simulink model "DYNctl_ver4_etud_obfusc"  (R2018b)
settings: Solver=ode45  StartTime=0.0  StopTime=tfin  FixedStep=0.001  RelTol=1e-09  EnableMultiTasking=on
undefined symbols (not defined in the file or in its folder): Aplaque, Asphere, Bplaque, Bsphere, Cplaque, Csphere, Dplaque, Dsphere, invTDEF
settings Model: Creator=delafontaine  LastModifiedBy=Vincent
settings DataIOCC: LimitDataPoints=on  SaveFormat=Array  SignalLoggingSaveFormat=ModelDataLogs
settings OptimizationCC: LifeSpan=inf
settings DebuggingCC: UnderspecifiedInitializationDetection=Classic  MergeDetectMultiDrivingBlocksExec=none  MultiTaskDSMMsg=warning  MultiTaskCondExecSysMsg=none  SFUnexpectedBacktrackingDiag=warning  SFNoUnconditionalDefaultTransitionDiag=warning  SFExecutionAtInitializationDiag=none
settings HardwareCC: ProdBitPerPointer=32  ProdBitPerSizeT=32  ProdBitPerPtrDiffT=32  ProdLargestAtomicFloat=None  ProdIntDivRoundTo=Undefined  ProdEndianess=Unspecified  ProdWordSize=32  ProdHWDeviceType=32-bit Generic
settings ModelReferenceCC: PropagateSignalLabelsOutOfModel=off
settings SFSimCC: SimUseLocalCustomCode=off
settings RTWCC: RTWUseLocalCustomCode=off
settings CodeAppCC: StateflowObjectComments=on
settings GRTTargetCC: TargetLangStandard=C89/C90 (ANSI)  GeneratePreprocessorConditionals=Disable all
settings ConfigComp: CovMetricSettings=dw  CovHtmlReporting=on  CovSaveCumulativeToWorkspaceVar=on  CovSaveSingleToWorkspaceVar=on  CovExternalEMLEnable=off  CovSFcnEnable=off

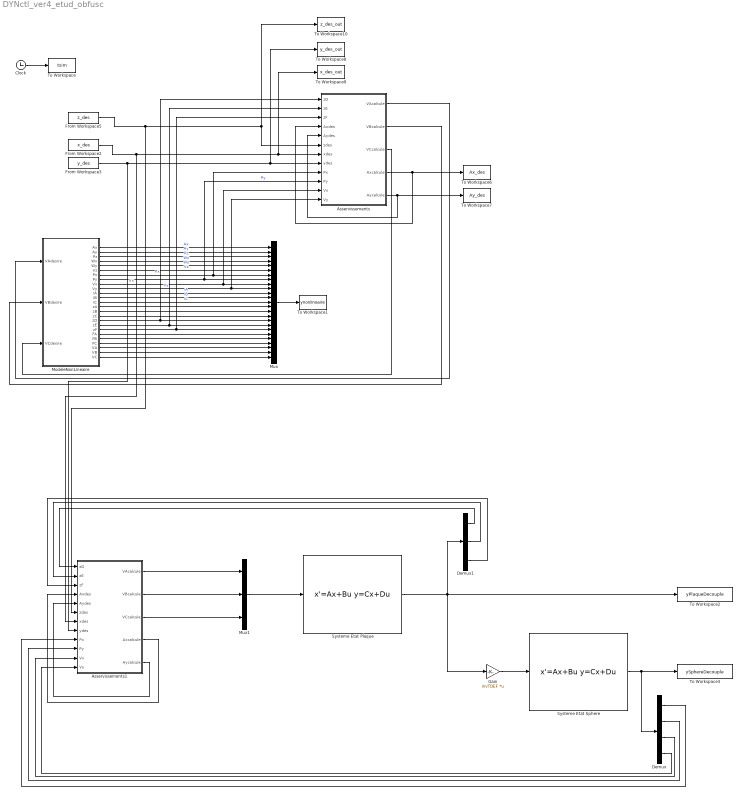
== system DYNctl_ver4_etud_obfusc ==
  Asservissements : Subsystem
      mask help: Simulink:masks:GenSFuncDesc_MD
      mask Help: eval('feval(''rtwprivate'',''rtwhelpview'',''rtw_sfcn_block'')');
  Asservissements1 : Subsystem
      mask help: Simulink:masks:GenSFuncDesc_MD
      mask Help: eval('feval(''rtwprivate'',''rtwhelpview'',''rtw_sfcn_block'')');
  Clock : Clock
  Demux : Demux
  Demux1 : Demux  Outputs=3
  From Workspace2 : FromWorkspace  VariableName=x_des  SampleTime=0  Interpolate=off  OutputAfterFinalValue=Holding final value
  From Workspace3 : FromWorkspace  VariableName=y_des  SampleTime=0  Interpolate=off  OutputAfterFinalValue=Holding final value
  From Workspace5 : FromWorkspace  VariableName=z_des  SampleTime=0  Interpolate=off  OutputAfterFinalValue=Holding final value
  Gain : Gain  Gain=invTDEF  Multiplication=Matrix(K*u)
  ModeleNonLineaire : Subsystem
      mask help: Simulink:masks:GenSFuncDesc_MD
      mask Help: eval('feval(''rtwprivate'',''rtwhelpview'',''rtw_sfcn_block'')');
  Mux : Mux  Inputs=25
  Mux1 : Mux  Inputs=3
  Systeme Etat Plaque : StateSpace  A=Aplaque  B=Bplaque  C=Cplaque  D=Dplaque  InitialCondition=0
  Systeme Etat Sphere : StateSpace  A=Asphere  B=Bsphere  C=Csphere  D=Dsphere  InitialCondition=0
  To Workspace : ToWorkspace  VariableName=tsim  SampleTime=-1
  To Workspace1 : ToWorkspace  VariableName=ynonlineaire  SampleTime=-1
  To Workspace10 : ToWorkspace  VariableName=z_des_out  SampleTime=-1
  To Workspace2 : ToWorkspace  VariableName=yPlaqueDecouple  SaveFormat=Timeseries  SampleTime=-1
  To Workspace3 : ToWorkspace  VariableName=ySphereDecouple  SaveFormat=Timeseries  SampleTime=-1
  To Workspace6 : ToWorkspace  VariableName=Ax_des  SampleTime=-1
  To Workspace7 : ToWorkspace  VariableName=Ay_des  SampleTime=-1
  To Workspace8 : ToWorkspace  VariableName=y_des_out  SampleTime=-1
  To Workspace9 : ToWorkspace  VariableName=x_des_out  SampleTime=-1
  wires:
  Mux/1 -> To Workspace1/1
  Clock/1 -> To Workspace/1
  From Workspace5/1 -> Asservissements1/6(zdes), Asservissements/6(zdes), To Workspace10/1
  ModeleNonLineaire/1(Ax) -> Mux/1  "Ax"
  ModeleNonLineaire/2(Ay) -> Mux/2  "Ay"
  ModeleNonLineaire/3(Pz) -> Mux/3  "Pz"
  ModeleNonLineaire/4(Wx) -> Mux/4  "Wx"
  ModeleNonLineaire/5(Wy) -> Mux/5  "Wy"
  ModeleNonLineaire/6(Vz) -> Mux/6  "Vz"
  ModeleNonLineaire/7(Px) -> Asservissements/9(Px), Mux/7  "Px"
  ModeleNonLineaire/8(Py) -> Asservissements/10(Py), Mux/8  "Py"
  ModeleNonLineaire/9(Vx) -> Asservissements/11(Vx), Mux/9  "Vx"
  ModeleNonLineaire/10(Vy) -> Asservissements/12(Vy), Mux/10  "Vy"
  ModeleNonLineaire/11(IA) -> Mux/11  "IA"
  ModeleNonLineaire/12(IB) -> Mux/12  "IB"
  ModeleNonLineaire/13(IC) -> Mux/13  "IC"
  From Workspace3/1 -> Asservissements1/8(ydes), Asservissements/8(ydes), To Workspace8/1
  From Workspace2/1 -> Asservissements1/7(xdes), Asservissements/7(xdes), To Workspace9/1
  ModeleNonLineaire/20(FA) -> Mux/20
  ModeleNonLineaire/21(FB) -> Mux/21
  ModeleNonLineaire/22(FC) -> Mux/22
  ModeleNonLineaire/23(VA) -> Mux/23
  ModeleNonLineaire/24(VB) -> Mux/24
  ModeleNonLineaire/25(VC) -> Mux/25
  ModeleNonLineaire/17(zD) -> Asservissements/1(zD), Mux/17
  ModeleNonLineaire/18(zE) -> Asservissements/2(zE), Mux/18
  ModeleNonLineaire/19(zF) -> Asservissements/3(zF), Mux/19
  ModeleNonLineaire/14(zA) -> Mux/14
  ModeleNonLineaire/15(zB) -> Mux/15
  ModeleNonLineaire/16(zC) -> Mux/16
  Asservissements/4(Axcalcule) -> Asservissements/4(Axdes), To Workspace6/1
  Asservissements/5(Aycalcule) -> Asservissements/5(Aydes), To Workspace7/1
  Asservissements/1(VAcalcule) -> ModeleNonLineaire/1(VAdesire)
  Asservissements/2(VBcalcule) -> ModeleNonLineaire/2(VBdesire)
  Mux1/1 -> Systeme Etat Plaque/1
  Systeme Etat Plaque/1 -> Demux1/1, Gain/1, To Workspace2/1
  Asservissements/3(VCcalcule) -> ModeleNonLineaire/3(VCdesire)
  Asservissements1/1(VAcalcule) -> Mux1/1
  Asservissements1/2(VBcalcule) -> Mux1/2
  Asservissements1/3(VCcalcule) -> Mux1/3
  Asservissements1/4(Axcalcule) -> Asservissements1/4(Axdes)
  Asservissements1/5(Aycalcule) -> Asservissements1/5(Aydes)
  Gain/1 -> Systeme Etat Sphere/1
  Systeme Etat Sphere/1 -> To Workspace3/1, Demux/1
  Demux/1 -> Asservissements1/9(Px)
  Demux/2 -> Asservissements1/10(Py)
  Demux/3 -> Asservissements1/11(Vx)
  Demux/4 -> Asservissements1/12(Vy)
  Demux1/1 -> Asservissements1/1(zD)
  Demux1/2 -> Asservissements1/2(zE)
  Demux1/3 -> Asservissements1/3(zF)

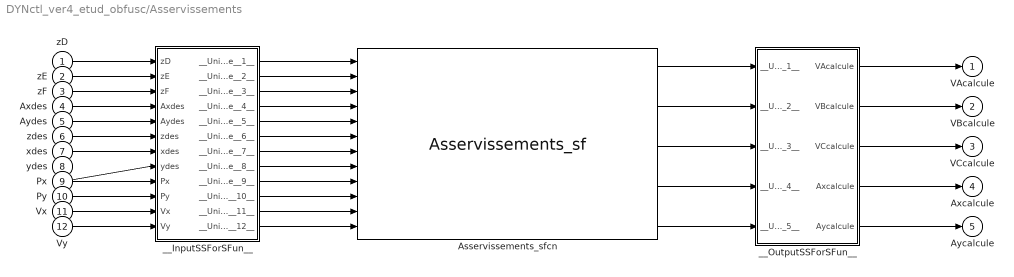
== system DYNctl_ver4_etud_obfusc/Asservissements ==
  zD : Inport
  zE : Inport  Port=2
  zF : Inport  Port=3
  Axdes : Inport  Port=4
  Aydes : Inport  Port=5
  zdes : Inport  Port=6
  xdes : Inport  Port=7
  ydes : Inport  Port=8
  Px : Inport  Port=9
  Py : Inport  Port=10
  Vx : Inport  Port=11
  Vy : Inport  Port=12
  Asservissements_sfcn : S-Function  FunctionName=Asservissements_sf  SFunctionModules=""  SFunctionDeploymentMode=off  EnableBusSupport=off  mask{rtw_sf_name=Asservissements_sf, showVar=off}
      mask prompts: rtw_sf_name "Simulink:masks:GenSFuncName_MP"; showVar "Simulink:masks:GenSFuncShowModuleList_MP"
      mask help: Simulink:masks:GenSFuncDesc_MD
      mask init:
      | displist = '';
      | if ~strcmp(get_param(gcb, 'FunctionName'), rtw_sf_name);
      |   set_param(gcb, 'FunctionName', rtw_sf_name);
      | end
      | % Check if we are generating code
      | rtw_mode = false;
      | if strcmpi(get_param(bdroot(gcb),'SimulationStatus'),'Initializing')
      | 	rtw_mode = strcmpi(get_param(bdroot(gcb),'BuildingRTWCode'),'on') && ...
      | 		~strcmpi(get_param(bdroot(gcb),'TargetStyle'),'SimulationTarget');
      | end
      | if showVar || rtw_mode
      | 	if exist('rtwsfunc') == 2 | exist('rtwsfunc') == 6
      | 		tmplist = rtwsfunc(rtw_sf_name,gcb);
      | 		tmplist = DAStudio.message('Simulink:masks:GenSFuncListOfModules_IC', tmplist);
      | 	elseif showVar
      | 		tmplist1 = DAStudio.message('Simulink:masks:GenSFuncListOfModules_IC', '');
      |         tmplist2 = DAStudio.message('Simulink:masks:GenSFuncNotLicensed_IC');
      |         tmplist = [tmplist1 tmplist2];
      |  	end
      | end
      | if showVar
      |   displist = tmplist;
      | end
      settings: CopyFcn=|
      | if ~strcmp(get_param(gcb,'Linkstatus'),'none') && ...
      | ~strcmp(get_param(gcb,'Linkstatus'),'implicit')
      |   set_param(gcb,'LinkStatus','none');
      | end
      mask Help: eval('feval(''rtwprivate'',''rtwhelpview'',''rtw_sfcn_block'')');
      mask Display:
      | port_label('input',1,'zD');
      | port_label('input',2,'zE');
      | port_label('input',3,'zF');
      | port_label('input',4,'Axdes');
      | port_label('input',5,'Aydes');
      | port_label('input',6,'zdes');
      | port_label('input',7,'xdes');
      | port_label('input',8,'ydes');
      | port_label('input',9,'Px');
      | port_label('input',10,'Py');
      | port_label('input',11,'Vx');
      | port_label('input',12,'Vy');
      | port_label('output',1,'VAcalcule');
      | port_label('output',2,'VBcalcule');
      | port_label('output',3,'VCcalcule');
      | port_label('output',4,'Axcalcule');
      | port_label('output',5,'Aycalcule');
  __InputSSForSFun__ : Subsystem
  __OutputSSForSFun__ : Subsystem
  VAcalcule : Outport
  VBcalcule : Outport  Port=2
  VCcalcule : Outport  Port=3
  Axcalcule : Outport  Port=4
  Aycalcule : Outport  Port=5
  wires:
  zD/1 -> __InputSSForSFun__/1(zD)
  zE/1 -> __InputSSForSFun__/2(zE)
  zF/1 -> __InputSSForSFun__/3(zF)
  Axdes/1 -> __InputSSForSFun__/4(Axdes)
  Aydes/1 -> __InputSSForSFun__/5(Aydes)
  zdes/1 -> __InputSSForSFun__/6(zdes)
  xdes/1 -> __InputSSForSFun__/7(xdes)
  ydes/1 -> __InputSSForSFun__/8(ydes)
  Px/1 -> __InputSSForSFun__/9(Px)
  Py/1 -> __InputSSForSFun__/10(Py)
  Vx/1 -> __InputSSForSFun__/11(Vx)
  Vy/1 -> __InputSSForSFun__/12(Vy)
  __InputSSForSFun__/1(__UniqueOutportName__1__) -> Asservissements_sfcn/1
  __InputSSForSFun__/2(__UniqueOutportName__2__) -> Asservissements_sfcn/2
  __InputSSForSFun__/3(__UniqueOutportName__3__) -> Asservissements_sfcn/3
  __InputSSForSFun__/4(__UniqueOutportName__4__) -> Asservissements_sfcn/4
  __InputSSForSFun__/5(__UniqueOutportName__5__) -> Asservissements_sfcn/5
  __InputSSForSFun__/6(__UniqueOutportName__6__) -> Asservissements_sfcn/6
  __InputSSForSFun__/7(__UniqueOutportName__7__) -> Asservissements_sfcn/7
  __InputSSForSFun__/8(__UniqueOutportName__8__) -> Asservissements_sfcn/8
  __InputSSForSFun__/9(__UniqueOutportName__9__) -> Asservissements_sfcn/9
  __InputSSForSFun__/10(__UniqueOutportName__10__) -> Asservissements_sfcn/10
  __InputSSForSFun__/11(__UniqueOutportName__11__) -> Asservissements_sfcn/11
  __InputSSForSFun__/12(__UniqueOutportName__12__) -> Asservissements_sfcn/12
  Asservissements_sfcn/1 -> __OutputSSForSFun__/1(__UniqueInportName__1__)
  Asservissements_sfcn/2 -> __OutputSSForSFun__/2(__UniqueInportName__2__)
  Asservissements_sfcn/3 -> __OutputSSForSFun__/3(__UniqueInportName__3__)
  Asservissements_sfcn/4 -> __OutputSSForSFun__/4(__UniqueInportName__4__)
  Asservissements_sfcn/5 -> __OutputSSForSFun__/5(__UniqueInportName__5__)
  __OutputSSForSFun__/1(VAcalcule) -> VAcalcule/1
  __OutputSSForSFun__/2(VBcalcule) -> VBcalcule/1
  __OutputSSForSFun__/3(VCcalcule) -> VCcalcule/1
  __OutputSSForSFun__/4(Axcalcule) -> Axcalcule/1
  __OutputSSForSFun__/5(Aycalcule) -> Aycalcule/1

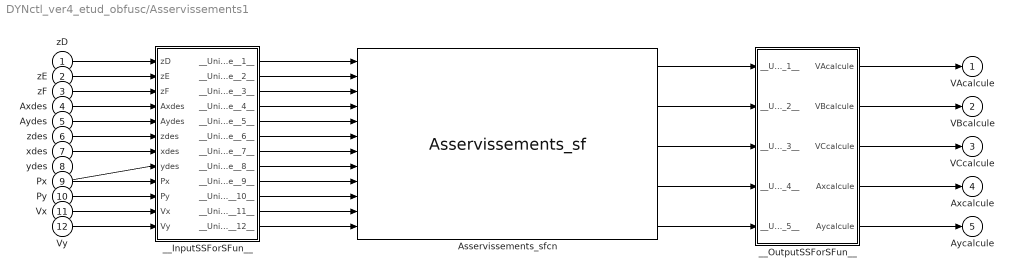
== system DYNctl_ver4_etud_obfusc/Asservissements1 ==
  zD : Inport
  zE : Inport  Port=2
  zF : Inport  Port=3
  Axdes : Inport  Port=4
  Aydes : Inport  Port=5
  zdes : Inport  Port=6
  xdes : Inport  Port=7
  ydes : Inport  Port=8
  Px : Inport  Port=9
  Py : Inport  Port=10
  Vx : Inport  Port=11
  Vy : Inport  Port=12
  Asservissements_sfcn : S-Function  FunctionName=Asservissements_sf  SFunctionModules=""  SFunctionDeploymentMode=off  EnableBusSupport=off  mask{rtw_sf_name=Asservissements_sf, showVar=off}
      mask prompts: rtw_sf_name "Simulink:masks:GenSFuncName_MP"; showVar "Simulink:masks:GenSFuncShowModuleList_MP"
      mask help: Simulink:masks:GenSFuncDesc_MD
      mask init: same as DYNctl_ver4_etud_obfusc/Asservissements/Asservissements_sfcn
      settings: CopyFcn=|
      | if ~strcmp(get_param(gcb,'Linkstatus'),'none') && ...
      | ~strcmp(get_param(gcb,'Linkstatus'),'implicit')
      |   set_param(gcb,'LinkStatus','none');
      | end
      mask Help: eval('feval(''rtwprivate'',''rtwhelpview'',''rtw_sfcn_block'')');
      mask Display:
      | port_label('input',1,'zD');
      | port_label('input',2,'zE');
      | port_label('input',3,'zF');
      | port_label('input',4,'Axdes');
      | port_label('input',5,'Aydes');
      | port_label('input',6,'zdes');
      | port_label('input',7,'xdes');
      | port_label('input',8,'ydes');
      | port_label('input',9,'Px');
      | port_label('input',10,'Py');
      | port_label('input',11,'Vx');
      | port_label('input',12,'Vy');
      | port_label('output',1,'VAcalcule');
      | port_label('output',2,'VBcalcule');
      | port_label('output',3,'VCcalcule');
      | port_label('output',4,'Axcalcule');
      | port_label('output',5,'Aycalcule');
  __InputSSForSFun__ : Subsystem
  __OutputSSForSFun__ : Subsystem
  VAcalcule : Outport
  VBcalcule : Outport  Port=2
  VCcalcule : Outport  Port=3
  Axcalcule : Outport  Port=4
  Aycalcule : Outport  Port=5
  wires:
  zD/1 -> __InputSSForSFun__/1(zD)
  zE/1 -> __InputSSForSFun__/2(zE)
  zF/1 -> __InputSSForSFun__/3(zF)
  Axdes/1 -> __InputSSForSFun__/4(Axdes)
  Aydes/1 -> __InputSSForSFun__/5(Aydes)
  zdes/1 -> __InputSSForSFun__/6(zdes)
  xdes/1 -> __InputSSForSFun__/7(xdes)
  ydes/1 -> __InputSSForSFun__/8(ydes)
  Px/1 -> __InputSSForSFun__/9(Px)
  Py/1 -> __InputSSForSFun__/10(Py)
  Vx/1 -> __InputSSForSFun__/11(Vx)
  Vy/1 -> __InputSSForSFun__/12(Vy)
  __InputSSForSFun__/1(__UniqueOutportName__1__) -> Asservissements_sfcn/1
  __InputSSForSFun__/2(__UniqueOutportName__2__) -> Asservissements_sfcn/2
  __InputSSForSFun__/3(__UniqueOutportName__3__) -> Asservissements_sfcn/3
  __InputSSForSFun__/4(__UniqueOutportName__4__) -> Asservissements_sfcn/4
  __InputSSForSFun__/5(__UniqueOutportName__5__) -> Asservissements_sfcn/5
  __InputSSForSFun__/6(__UniqueOutportName__6__) -> Asservissements_sfcn/6
  __InputSSForSFun__/7(__UniqueOutportName__7__) -> Asservissements_sfcn/7
  __InputSSForSFun__/8(__UniqueOutportName__8__) -> Asservissements_sfcn/8
  __InputSSForSFun__/9(__UniqueOutportName__9__) -> Asservissements_sfcn/9
  __InputSSForSFun__/10(__UniqueOutportName__10__) -> Asservissements_sfcn/10
  __InputSSForSFun__/11(__UniqueOutportName__11__) -> Asservissements_sfcn/11
  __InputSSForSFun__/12(__UniqueOutportName__12__) -> Asservissements_sfcn/12
  Asservissements_sfcn/1 -> __OutputSSForSFun__/1(__UniqueInportName__1__)
  Asservissements_sfcn/2 -> __OutputSSForSFun__/2(__UniqueInportName__2__)
  Asservissements_sfcn/3 -> __OutputSSForSFun__/3(__UniqueInportName__3__)
  Asservissements_sfcn/4 -> __OutputSSForSFun__/4(__UniqueInportName__4__)
  Asservissements_sfcn/5 -> __OutputSSForSFun__/5(__UniqueInportName__5__)
  __OutputSSForSFun__/1(VAcalcule) -> VAcalcule/1
  __OutputSSForSFun__/2(VBcalcule) -> VBcalcule/1
  __OutputSSForSFun__/3(VCcalcule) -> VCcalcule/1
  __OutputSSForSFun__/4(Axcalcule) -> Axcalcule/1
  __OutputSSForSFun__/5(Aycalcule) -> Aycalcule/1

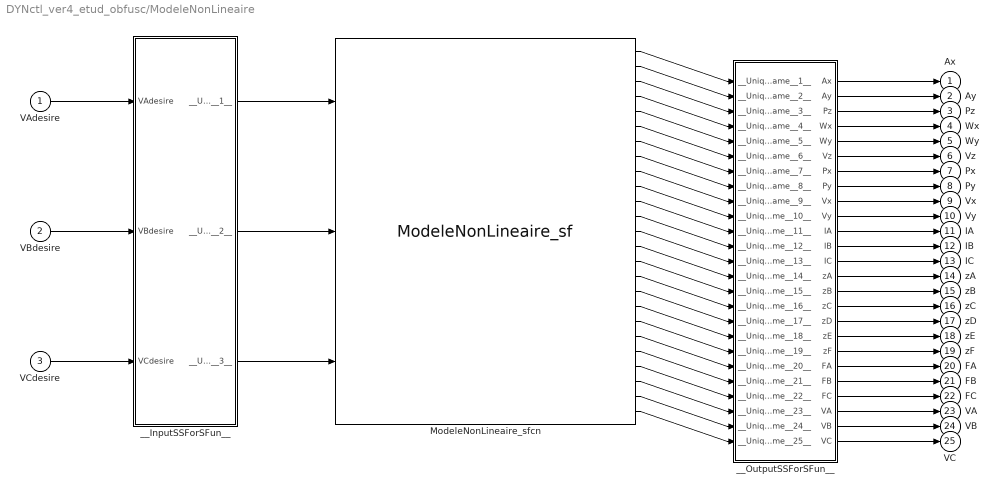
== system DYNctl_ver4_etud_obfusc/ModeleNonLineaire ==
  VAdesire : Inport
  VBdesire : Inport  Port=2
  VCdesire : Inport  Port=3
  ModeleNonLineaire_sfcn : S-Function  FunctionName=ModeleNonLineaire_sf  SFunctionModules=""  SFunctionDeploymentMode=off  EnableBusSupport=off  mask{rtw_sf_name=ModeleNonLineaire_sf, showVar=off}
      mask prompts: rtw_sf_name "Simulink:masks:GenSFuncName_MP"; showVar "Simulink:masks:GenSFuncShowModuleList_MP"
      mask help: Simulink:masks:GenSFuncDesc_MD
      mask init: same as DYNctl_ver4_etud_obfusc/Asservissements/Asservissements_sfcn
      settings: CopyFcn=|
      | if ~strcmp(get_param(gcb,'Linkstatus'),'none') && ...
      | ~strcmp(get_param(gcb,'Linkstatus'),'implicit')
      |   set_param(gcb,'LinkStatus','none');
      | end
      mask Help: eval('feval(''rtwprivate'',''rtwhelpview'',''rtw_sfcn_block'')');
      mask Display:
      | port_label('input',1,'VAdesire');
      | port_label('input',2,'VBdesire');
      | port_label('input',3,'VCdesire');
      | port_label('output',1,'Ax');
      | port_label('output',2,'Ay');
      | port_label('output',3,'Pz');
      | port_label('output',4,'Wx');
      | port_label('output',5,'Wy');
      | port_label('output',6,'Vz');
      | port_label('output',7,'Px');
      | port_label('output',8,'Py');
      | port_label('output',9,'Vx');
      | port_label('output',10,'Vy');
      | port_label('output',11,'IA');
      | port_label('output',12,'IB');
      | port_label('output',13,'IC');
      | port_label('output',14,'zA');
      | port_label('output',15,'zB');
      | port_label('output',16,'zC');
      | port_label('output',17,'zD');
      | port_label('output',18,'zE');
      | port_label('output',19,'zF');
      | port_label('output',20,'FA');
      | port_label('output',21,'FB');
      | port_label('output',22,'FC');
      | port_label('output',23,'VA');
      | port_label('output',24,'VB');
      | port_label('output',25,'VC');
  __InputSSForSFun__ : Subsystem
  __OutputSSForSFun__ : Subsystem
  Ax : Outport
  Ay : Outport  Port=2
  Pz : Outport  Port=3
  Wx : Outport  Port=4
  Wy : Outport  Port=5
  Vz : Outport  Port=6
  Px : Outport  Port=7
  Py : Outport  Port=8
  Vx : Outport  Port=9
  Vy : Outport  Port=10
  IA : Outport  Port=11
  IB : Outport  Port=12
  IC : Outport  Port=13
  zA : Outport  Port=14
  zB : Outport  Port=15
  zC : Outport  Port=16
  zD : Outport  Port=17
  zE : Outport  Port=18
  zF : Outport  Port=19
  FA : Outport  Port=20
  FB : Outport  Port=21
  FC : Outport  Port=22
  VA : Outport  Port=23
  VB : Outport  Port=24
  VC : Outport  Port=25
  wires:
  VAdesire/1 -> __InputSSForSFun__/1(VAdesire)
  VBdesire/1 -> __InputSSForSFun__/2(VBdesire)
  VCdesire/1 -> __InputSSForSFun__/3(VCdesire)
  __InputSSForSFun__/1(__UniqueOutportName__1__) -> ModeleNonLineaire_sfcn/1
  __InputSSForSFun__/2(__UniqueOutportName__2__) -> ModeleNonLineaire_sfcn/2
  __InputSSForSFun__/3(__UniqueOutportName__3__) -> ModeleNonLineaire_sfcn/3
  ModeleNonLineaire_sfcn/1 -> __OutputSSForSFun__/1(__UniqueInportName__1__)
  ModeleNonLineaire_sfcn/2 -> __OutputSSForSFun__/2(__UniqueInportName__2__)
  ModeleNonLineaire_sfcn/3 -> __OutputSSForSFun__/3(__UniqueInportName__3__)
  ModeleNonLineaire_sfcn/4 -> __OutputSSForSFun__/4(__UniqueInportName__4__)
  ModeleNonLineaire_sfcn/5 -> __OutputSSForSFun__/5(__UniqueInportName__5__)
  ModeleNonLineaire_sfcn/6 -> __OutputSSForSFun__/6(__UniqueInportName__6__)
  ModeleNonLineaire_sfcn/7 -> __OutputSSForSFun__/7(__UniqueInportName__7__)
  ModeleNonLineaire_sfcn/8 -> __OutputSSForSFun__/8(__UniqueInportName__8__)
  ModeleNonLineaire_sfcn/9 -> __OutputSSForSFun__/9(__UniqueInportName__9__)
  ModeleNonLineaire_sfcn/10 -> __OutputSSForSFun__/10(__UniqueInportName__10__)
  ModeleNonLineaire_sfcn/11 -> __OutputSSForSFun__/11(__UniqueInportName__11__)
  ModeleNonLineaire_sfcn/12 -> __OutputSSForSFun__/12(__UniqueInportName__12__)
  ModeleNonLineaire_sfcn/13 -> __OutputSSForSFun__/13(__UniqueInportName__13__)
  ModeleNonLineaire_sfcn/14 -> __OutputSSForSFun__/14(__UniqueInportName__14__)
  ModeleNonLineaire_sfcn/15 -> __OutputSSForSFun__/15(__UniqueInportName__15__)
  ModeleNonLineaire_sfcn/16 -> __OutputSSForSFun__/16(__UniqueInportName__16__)
  ModeleNonLineaire_sfcn/17 -> __OutputSSForSFun__/17(__UniqueInportName__17__)
  ModeleNonLineaire_sfcn/18 -> __OutputSSForSFun__/18(__UniqueInportName__18__)
  ModeleNonLineaire_sfcn/19 -> __OutputSSForSFun__/19(__UniqueInportName__19__)
  ModeleNonLineaire_sfcn/20 -> __OutputSSForSFun__/20(__UniqueInportName__20__)
  ModeleNonLineaire_sfcn/21 -> __OutputSSForSFun__/21(__UniqueInportName__21__)
  ModeleNonLineaire_sfcn/22 -> __OutputSSForSFun__/22(__UniqueInportName__22__)
  ModeleNonLineaire_sfcn/23 -> __OutputSSForSFun__/23(__UniqueInportName__23__)
  ModeleNonLineaire_sfcn/24 -> __OutputSSForSFun__/24(__UniqueInportName__24__)
  ModeleNonLineaire_sfcn/25 -> __OutputSSForSFun__/25(__UniqueInportName__25__)
  __OutputSSForSFun__/1(Ax) -> Ax/1
  __OutputSSForSFun__/2(Ay) -> Ay/1
  __OutputSSForSFun__/3(Pz) -> Pz/1
  __OutputSSForSFun__/4(Wx) -> Wx/1
  __OutputSSForSFun__/5(Wy) -> Wy/1
  __OutputSSForSFun__/6(Vz) -> Vz/1
  __OutputSSForSFun__/7(Px) -> Px/1
  __OutputSSForSFun__/8(Py) -> Py/1
  __OutputSSForSFun__/9(Vx) -> Vx/1
  __OutputSSForSFun__/10(Vy) -> Vy/1
  __OutputSSForSFun__/11(IA) -> IA/1
  __OutputSSForSFun__/12(IB) -> IB/1
  __OutputSSForSFun__/13(IC) -> IC/1
  __OutputSSForSFun__/14(zA) -> zA/1
  __OutputSSForSFun__/15(zB) -> zB/1
  __OutputSSForSFun__/16(zC) -> zC/1
  __OutputSSForSFun__/17(zD) -> zD/1
  __OutputSSForSFun__/18(zE) -> zE/1
  __OutputSSForSFun__/19(zF) -> zF/1
  __OutputSSForSFun__/20(FA) -> FA/1
  __OutputSSForSFun__/21(FB) -> FB/1
  __OutputSSForSFun__/22(FC) -> FC/1
  __OutputSSForSFun__/23(VA) -> VA/1
  __OutputSSForSFun__/24(VB) -> VB/1
  __OutputSSForSFun__/25(VC) -> VC/1

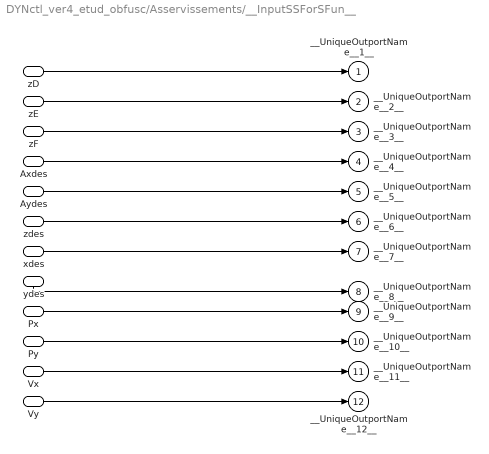
== system DYNctl_ver4_etud_obfusc/Asservissements/__InputSSForSFun__ ==
  zD : Inport
  zE : Inport  Port=2
  zF : Inport  Port=3
  Axdes : Inport  Port=4
  Aydes : Inport  Port=5
  zdes : Inport  Port=6
  xdes : Inport  Port=7
  ydes : Inport  Port=8
  Px : Inport  Port=9
  Py : Inport  Port=10
  Vx : Inport  Port=11
  Vy : Inport  Port=12
  __UniqueOutportName__1__ : Outport
  __UniqueOutportName__2__ : Outport  Port=2
  __UniqueOutportName__3__ : Outport  Port=3
  __UniqueOutportName__4__ : Outport  Port=4
  __UniqueOutportName__5__ : Outport  Port=5
  __UniqueOutportName__6__ : Outport  Port=6
  __UniqueOutportName__7__ : Outport  Port=7
  __UniqueOutportName__8__ : Outport  Port=8
  __UniqueOutportName__9__ : Outport  Port=9
  __UniqueOutportName__10__ : Outport  Port=10
  __UniqueOutportName__11__ : Outport  Port=11
  __UniqueOutportName__12__ : Outport  Port=12
  wires:
  zD/1 -> __UniqueOutportName__1__/1
  zE/1 -> __UniqueOutportName__2__/1
  zF/1 -> __UniqueOutportName__3__/1
  Axdes/1 -> __UniqueOutportName__4__/1
  Aydes/1 -> __UniqueOutportName__5__/1
  zdes/1 -> __UniqueOutportName__6__/1
  xdes/1 -> __UniqueOutportName__7__/1
  ydes/1 -> __UniqueOutportName__8__/1
  Px/1 -> __UniqueOutportName__9__/1
  Py/1 -> __UniqueOutportName__10__/1
  Vx/1 -> __UniqueOutportName__11__/1
  Vy/1 -> __UniqueOutportName__12__/1

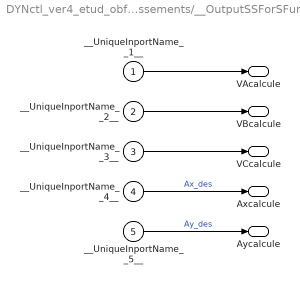
== system DYNctl_ver4_etud_obfusc/Asservissements/__OutputSSForSFun__ ==
  __UniqueInportName__1__ : Inport
  __UniqueInportName__2__ : Inport  Port=2
  __UniqueInportName__3__ : Inport  Port=3
  __UniqueInportName__4__ : Inport  Port=4
  __UniqueInportName__5__ : Inport  Port=5
  VAcalcule : Outport
  VBcalcule : Outport  Port=2
  VCcalcule : Outport  Port=3
  Axcalcule : Outport  Port=4
  Aycalcule : Outport  Port=5
  wires:
  __UniqueInportName__1__/1 -> VAcalcule/1
  __UniqueInportName__2__/1 -> VBcalcule/1
  __UniqueInportName__3__/1 -> VCcalcule/1
  __UniqueInportName__4__/1 -> Axcalcule/1  "Ax_des"
  __UniqueInportName__5__/1 -> Aycalcule/1  "Ay_des"

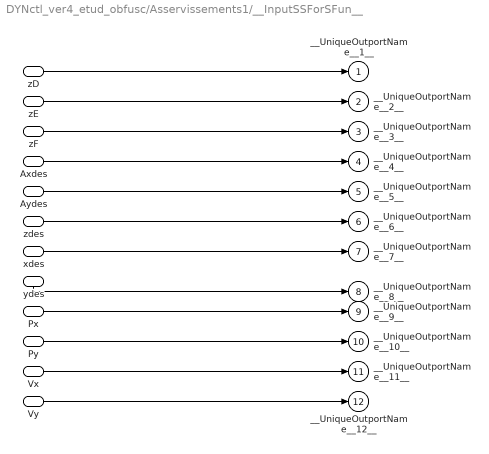
== system DYNctl_ver4_etud_obfusc/Asservissements1/__InputSSForSFun__ ==
  zD : Inport
  zE : Inport  Port=2
  zF : Inport  Port=3
  Axdes : Inport  Port=4
  Aydes : Inport  Port=5
  zdes : Inport  Port=6
  xdes : Inport  Port=7
  ydes : Inport  Port=8
  Px : Inport  Port=9
  Py : Inport  Port=10
  Vx : Inport  Port=11
  Vy : Inport  Port=12
  __UniqueOutportName__1__ : Outport
  __UniqueOutportName__2__ : Outport  Port=2
  __UniqueOutportName__3__ : Outport  Port=3
  __UniqueOutportName__4__ : Outport  Port=4
  __UniqueOutportName__5__ : Outport  Port=5
  __UniqueOutportName__6__ : Outport  Port=6
  __UniqueOutportName__7__ : Outport  Port=7
  __UniqueOutportName__8__ : Outport  Port=8
  __UniqueOutportName__9__ : Outport  Port=9
  __UniqueOutportName__10__ : Outport  Port=10
  __UniqueOutportName__11__ : Outport  Port=11
  __UniqueOutportName__12__ : Outport  Port=12
  wires:
  zD/1 -> __UniqueOutportName__1__/1
  zE/1 -> __UniqueOutportName__2__/1
  zF/1 -> __UniqueOutportName__3__/1
  Axdes/1 -> __UniqueOutportName__4__/1
  Aydes/1 -> __UniqueOutportName__5__/1
  zdes/1 -> __UniqueOutportName__6__/1
  xdes/1 -> __UniqueOutportName__7__/1
  ydes/1 -> __UniqueOutportName__8__/1
  Px/1 -> __UniqueOutportName__9__/1
  Py/1 -> __UniqueOutportName__10__/1
  Vx/1 -> __UniqueOutportName__11__/1
  Vy/1 -> __UniqueOutportName__12__/1

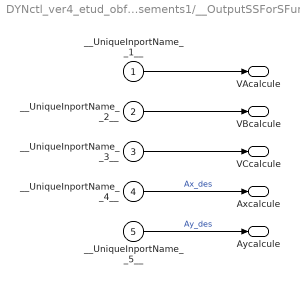
== system DYNctl_ver4_etud_obfusc/Asservissements1/__OutputSSForSFun__ ==
  __UniqueInportName__1__ : Inport
  __UniqueInportName__2__ : Inport  Port=2
  __UniqueInportName__3__ : Inport  Port=3
  __UniqueInportName__4__ : Inport  Port=4
  __UniqueInportName__5__ : Inport  Port=5
  VAcalcule : Outport
  VBcalcule : Outport  Port=2
  VCcalcule : Outport  Port=3
  Axcalcule : Outport  Port=4
  Aycalcule : Outport  Port=5
  wires:
  __UniqueInportName__1__/1 -> VAcalcule/1
  __UniqueInportName__2__/1 -> VBcalcule/1
  __UniqueInportName__3__/1 -> VCcalcule/1
  __UniqueInportName__4__/1 -> Axcalcule/1  "Ax_des"
  __UniqueInportName__5__/1 -> Aycalcule/1  "Ay_des"

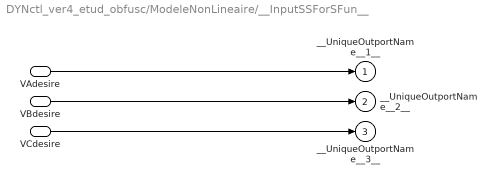
== system DYNctl_ver4_etud_obfusc/ModeleNonLineaire/__InputSSForSFun__ ==
  VAdesire : Inport
  VBdesire : Inport  Port=2
  VCdesire : Inport  Port=3
  __UniqueOutportName__1__ : Outport
  __UniqueOutportName__2__ : Outport  Port=2
  __UniqueOutportName__3__ : Outport  Port=3
  wires:
  VAdesire/1 -> __UniqueOutportName__1__/1
  VBdesire/1 -> __UniqueOutportName__2__/1
  VCdesire/1 -> __UniqueOutportName__3__/1

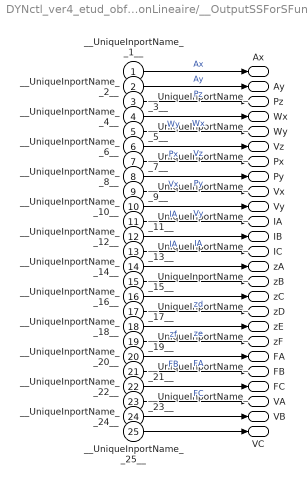
== system DYNctl_ver4_etud_obfusc/ModeleNonLineaire/__OutputSSForSFun__ ==
  __UniqueInportName__1__ : Inport
  __UniqueInportName__2__ : Inport  Port=2
  __UniqueInportName__3__ : Inport  Port=3
  __UniqueInportName__4__ : Inport  Port=4
  __UniqueInportName__5__ : Inport  Port=5
  __UniqueInportName__6__ : Inport  Port=6
  __UniqueInportName__7__ : Inport  Port=7
  __UniqueInportName__8__ : Inport  Port=8
  __UniqueInportName__9__ : Inport  Port=9
  __UniqueInportName__10__ : Inport  Port=10
  __UniqueInportName__11__ : Inport  Port=11
  __UniqueInportName__12__ : Inport  Port=12
  __UniqueInportName__13__ : Inport  Port=13
  __UniqueInportName__14__ : Inport  Port=14
  __UniqueInportName__15__ : Inport  Port=15
  __UniqueInportName__16__ : Inport  Port=16
  __UniqueInportName__17__ : Inport  Port=17
  __UniqueInportName__18__ : Inport  Port=18
  __UniqueInportName__19__ : Inport  Port=19
  __UniqueInportName__20__ : Inport  Port=20
  __UniqueInportName__21__ : Inport  Port=21
  __UniqueInportName__22__ : Inport  Port=22
  __UniqueInportName__23__ : Inport  Port=23
  __UniqueInportName__24__ : Inport  Port=24
  __UniqueInportName__25__ : Inport  Port=25
  Ax : Outport
  Ay : Outport  Port=2
  Pz : Outport  Port=3
  Wx : Outport  Port=4
  Wy : Outport  Port=5
  Vz : Outport  Port=6
  Px : Outport  Port=7
  Py : Outport  Port=8
  Vx : Outport  Port=9
  Vy : Outport  Port=10
  IA : Outport  Port=11
  IB : Outport  Port=12
  IC : Outport  Port=13
  zA : Outport  Port=14
  zB : Outport  Port=15
  zC : Outport  Port=16
  zD : Outport  Port=17
  zE : Outport  Port=18
  zF : Outport  Port=19
  FA : Outport  Port=20
  FB : Outport  Port=21
  FC : Outport  Port=22
  VA : Outport  Port=23
  VB : Outport  Port=24
  VC : Outport  Port=25
  wires:
  __UniqueInportName__1__/1 -> Ax/1  "Ax"
  __UniqueInportName__2__/1 -> Ay/1  "Ay"
  __UniqueInportName__3__/1 -> Pz/1  "Pz"
  __UniqueInportName__4__/1 -> Wx/1  "Wx"
  __UniqueInportName__5__/1 -> Wy/1  "Wy"
  __UniqueInportName__6__/1 -> Vz/1  "Vz"
  __UniqueInportName__7__/1 -> Px/1  "Px"
  __UniqueInportName__8__/1 -> Py/1  "Py"
  __UniqueInportName__9__/1 -> Vx/1  "Vx"
  __UniqueInportName__10__/1 -> Vy/1  "Vy"
  __UniqueInportName__11__/1 -> IA/1  "IA"
  __UniqueInportName__12__/1 -> IB/1  "IA"
  __UniqueInportName__13__/1 -> IC/1  "IA"
  __UniqueInportName__14__/1 -> zA/1
  __UniqueInportName__15__/1 -> zB/1
  __UniqueInportName__16__/1 -> zC/1
  __UniqueInportName__17__/1 -> zD/1  "zd"
  __UniqueInportName__18__/1 -> zE/1  "ze"
  __UniqueInportName__19__/1 -> zF/1  "zf"
  __UniqueInportName__20__/1 -> FA/1  "FA"
  __UniqueInportName__21__/1 -> FB/1  "FB"
  __UniqueInportName__22__/1 -> FC/1  "FC"
  __UniqueInportName__23__/1 -> VA/1
  __UniqueInportName__24__/1 -> VB/1
  __UniqueInportName__25__/1 -> VC/1
